simulink model "continuous"  (R2023b)
settings: Solver=FixedStepAuto  StartTime=0.0  StopTime=5  FixedStep=0.01  RelTol=1e-3
InitFcn:
  | clc;clear
  | close all
  | g = [0;2.092];
  | k1 = [-141.9203 -4.5243];
  | k2 = [-101.5134 -3.1941];
  | x0 = [0.4;-10];
settings Model: Creator=IHC  LastModifiedBy=IHC

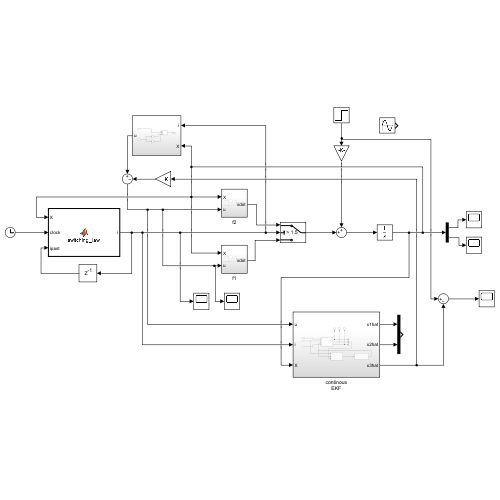
[thumbnail: Simulink's stored preview of the top-level diagram]
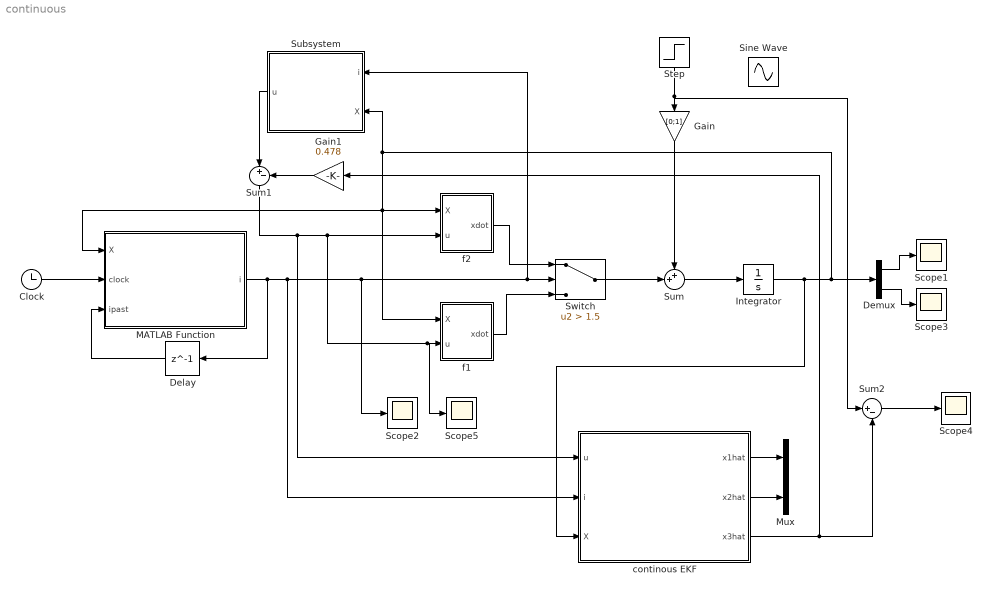
== system continuous ==
  Clock : Clock
  Delay : Delay  DelayLength=1  InitialCondition=2
  Demux : Demux  Outputs=2
  Gain : Gain  Gain=[0;1]
  Gain1 : Gain  Gain=0.478
  Integrator : Integrator  InitialCondition=x0
  MATLAB Function : MATLAB Function  TreatAsAtomicUnit=on
  Mux : Mux  Inputs=2
  Scope{1..5} (5 alike) : Scope
  Sine Wave : Sin  SampleTime=0
  Step : Step  Time=0  After=4  SampleTime=0
  Subsystem : Subsystem
  Sum : Sum  Inputs=++|
  Sum1 : Sum  Inputs=|+-
  Sum2 : Sum  Inputs=|+-
  Switch : Switch  Criteria=u2 > Threshold  Threshold=1.5  SaturateOnIntegerOverflow=off  InputSameDT=off
  continous EKF : Subsystem
  f1 : Subsystem
  f2 : Subsystem
  wires:
  Clock/1 -> MATLAB Function/2(clock)
  Subsystem/1(u) -> Sum1/1
  Demux/1 -> Scope1/1
  Demux/2 -> Scope3/1
  Delay/1 -> MATLAB Function/3(ipast)
  MATLAB Function/1(i) -> Delay/1, continous EKF/2(i), Scope2/1, Subsystem/1(i), Switch/2
  f2/1(xdot) -> Switch/1
  f1/1(xdot) -> Switch/3
  Switch/1 -> Sum/2
  Sum/1 -> Integrator/1
  Gain/1 -> Sum/1
  Step/1 -> Sum2/1, Gain/1
  Integrator/1 -> continous EKF/3(X), Demux/1, MATLAB Function/1(X), f1/1(X), f2/1(X), Subsystem/2(X)
  Sum1/1 -> continous EKF/1(u), Scope5/1, f1/2(u), f2/2(u)
  Sum2/1 -> Scope4/1
  Gain1/1 -> Sum1/2
  continous EKF/3(x3hat) -> Gain1/1, Sum2/2
  continous EKF/1(x1hat) -> Mux/1
  continous EKF/2(x2hat) -> Mux/2

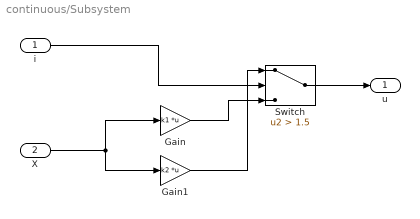
== system continuous/Subsystem ==
  i : Inport
  X : Inport  Port=2
  Gain : Gain  Gain=k1  Multiplication=Matrix(K*u)
  Gain1 : Gain  Gain=k2  Multiplication=Matrix(K*u)
  Switch : Switch  Criteria=u2 > Threshold  Threshold=1.5  SaturateOnIntegerOverflow=off  InputSameDT=off
  u : Outport
  wires:
  Switch/1 -> u/1
  i/1 -> Switch/2
  X/1 -> Gain1/1, Gain/1
  Gain/1 -> Switch/3
  Gain1/1 -> Switch/1

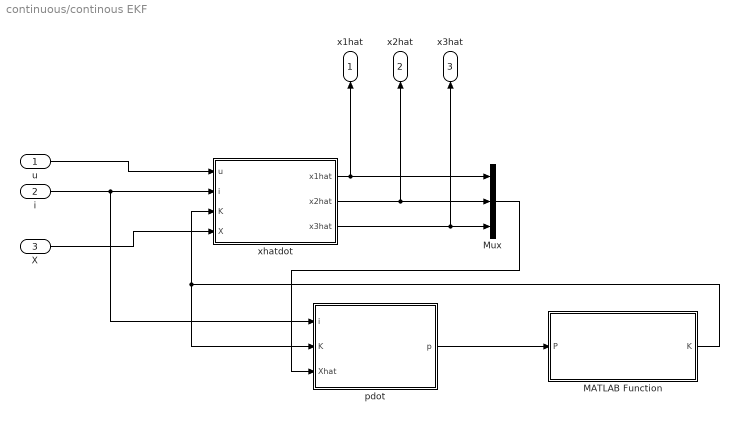
== system continuous/continous EKF ==
  u : Inport
  i : Inport  Port=2
  X : Inport  Port=3
  MATLAB Function : MATLAB Function  TreatAsAtomicUnit=on
  Mux : Mux  Inputs=3
  pdot : Subsystem
  xhatdot : Subsystem
  x1hat : Outport
  x2hat : Outport  Port=2
  x3hat : Outport  Port=3
  wires:
  u/1 -> xhatdot/1(u)
  i/1 -> pdot/1(i), xhatdot/2(i)
  xhatdot/1(x1hat) -> Mux/1, x1hat/1
  xhatdot/2(x2hat) -> Mux/2, x2hat/1
  xhatdot/3(x3hat) -> Mux/3, x3hat/1
  X/1 -> xhatdot/4(X)
  MATLAB Function/1(K) -> pdot/2(K), xhatdot/3(K)
  Mux/1 -> pdot/3(Xhat)
  pdot/1(p) -> MATLAB Function/1(P)

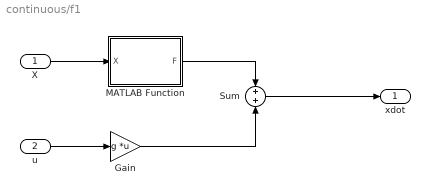
== system continuous/f1 ==
  X : Inport
  u : Inport  Port=2
  Gain : Gain  Gain=g  Multiplication=Matrix(K*u)
  MATLAB Function : MATLAB Function  TreatAsAtomicUnit=on
  Sum : Sum
  xdot : Outport
  wires:
  u/1 -> Gain/1
  X/1 -> MATLAB Function/1(X)
  Gain/1 -> Sum/2
  MATLAB Function/1(F) -> Sum/1
  Sum/1 -> xdot/1

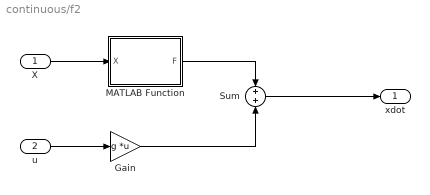
== system continuous/f2 ==
  X : Inport
  u : Inport  Port=2
  Gain : Gain  Gain=g  Multiplication=Matrix(K*u)
  MATLAB Function : MATLAB Function  TreatAsAtomicUnit=on
  Sum : Sum
  xdot : Outport
  wires:
  Sum/1 -> xdot/1
  u/1 -> Gain/1
  MATLAB Function/1(F) -> Sum/1
  Gain/1 -> Sum/2
  X/1 -> MATLAB Function/1(X)

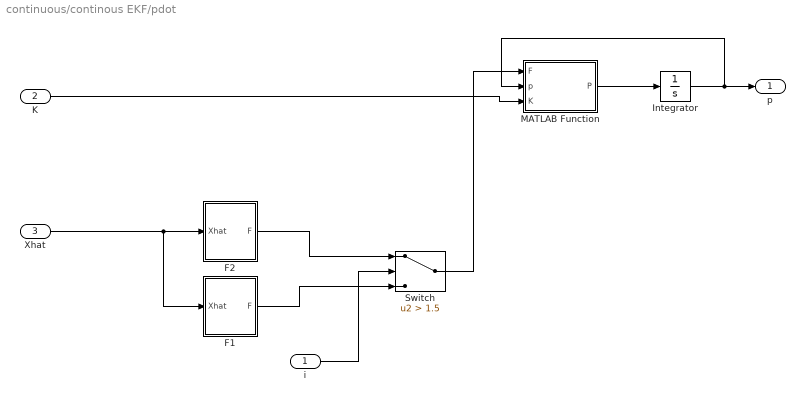
== system continuous/continous EKF/pdot ==
  i : Inport
  K : Inport  Port=2
  Xhat : Inport  Port=3
  F1 : Subsystem
  F2 : Subsystem
  Integrator : Integrator  InitialCondition=diag([0.001,0.001,10])
  MATLAB Function : MATLAB Function  TreatAsAtomicUnit=on
  Switch : Switch  Criteria=u2 > Threshold  Threshold=1.5  SaturateOnIntegerOverflow=off  InputSameDT=off
  p : Outport
  wires:
  F2/1(F) -> Switch/1
  i/1 -> Switch/2
  Integrator/1 -> MATLAB Function/2(p), p/1
  Xhat/1 -> F1/1(Xhat), F2/1(Xhat)
  F1/1(F) -> Switch/3
  MATLAB Function/1(P) -> Integrator/1
  Switch/1 -> MATLAB Function/1(F)
  K/1 -> MATLAB Function/3(K)

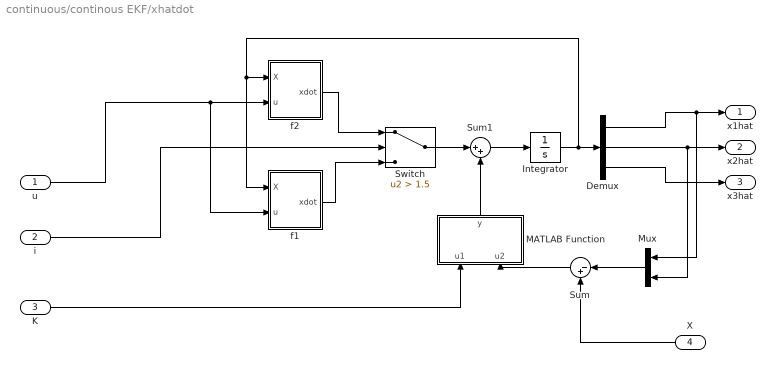
== system continuous/continous EKF/xhatdot ==
  u : Inport
  i : Inport  Port=2
  K : Inport  Port=3
  X : Inport  Port=4
  Demux : Demux  Outputs=3
  Integrator : Integrator  InitialCondition=[x0;0]
  MATLAB Function : MATLAB Function  TreatAsAtomicUnit=on
  Mux : Mux  Inputs=2
  Sum : Sum  Inputs=|-+
  Sum1 : Sum  Inputs=|++
  Switch : Switch  Criteria=u2 > Threshold  Threshold=1.5  SaturateOnIntegerOverflow=off  InputSameDT=off
  f1 : Subsystem
  f2 : Subsystem
  x1hat : Outport
  x2hat : Outport  Port=2
  x3hat : Outport  Port=3
  wires:
  Demux/2 -> Mux/2, x2hat/1
  Demux/3 -> x3hat/1
  f1/1(xdot) -> Switch/3
  f2/1(xdot) -> Switch/1
  u/1 -> f1/2(u), f2/2(u)
  i/1 -> Switch/2
  Demux/1 -> Mux/1, x1hat/1
  Integrator/1 -> f1/1(X), f2/1(X), Demux/1
  Switch/1 -> Sum1/1
  Sum1/1 -> Integrator/1
  X/1 -> Sum/2
  Mux/1 -> Sum/1
  MATLAB Function/1(y) -> Sum1/2
  Sum/1 -> MATLAB Function/2(u2)
  K/1 -> MATLAB Function/1(u1)

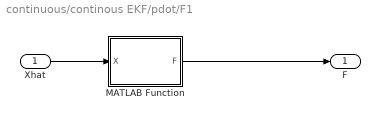
== system continuous/continous EKF/pdot/F1 ==
  Xhat : Inport
  MATLAB Function : MATLAB Function  TreatAsAtomicUnit=on
  F : Outport
  wires:
  Xhat/1 -> MATLAB Function/1(X)
  MATLAB Function/1(F) -> F/1

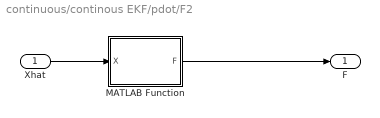
== system continuous/continous EKF/pdot/F2 ==
  Xhat : Inport
  MATLAB Function : MATLAB Function  TreatAsAtomicUnit=on
  F : Outport
  wires:
  Xhat/1 -> MATLAB Function/1(X)
  MATLAB Function/1(F) -> F/1

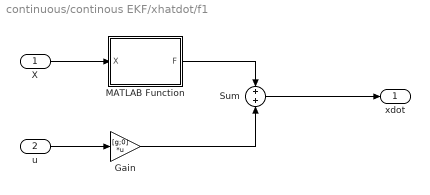
== system continuous/continous EKF/xhatdot/f1 ==
  X : Inport
  u : Inport  Port=2
  Gain : Gain  Gain=[g;0]  Multiplication=Matrix(K*u)
  MATLAB Function : MATLAB Function  TreatAsAtomicUnit=on
  Sum : Sum
  xdot : Outport
  wires:
  u/1 -> Gain/1
  X/1 -> MATLAB Function/1(X)
  Gain/1 -> Sum/2
  MATLAB Function/1(F) -> Sum/1
  Sum/1 -> xdot/1

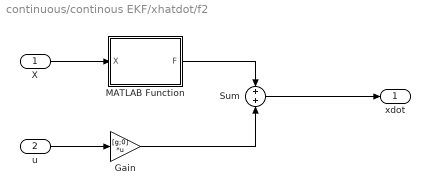
== system continuous/continous EKF/xhatdot/f2 ==
  X : Inport
  u : Inport  Port=2
  Gain : Gain  Gain=[g;0]  Multiplication=Matrix(K*u)
  MATLAB Function : MATLAB Function  TreatAsAtomicUnit=on
  Sum : Sum
  xdot : Outport
  wires:
  Sum/1 -> xdot/1
  u/1 -> Gain/1
  MATLAB Function/1(F) -> Sum/1
  Gain/1 -> Sum/2
  X/1 -> MATLAB Function/1(X)

== matlab function continuous/f2/MATLAB Function ==
  data: X input; F output
function F = fcn(X)
x1 = X(1);
x2 = X(2);
alpha = -7.2*10^10*(x1+0.5)*exp(-8750/(x2+350))+0.5;
beta = 1.506*10^13*(x1+0.5)*exp(-8750/(x2+350))-104.6;
f1=-2*x1+alpha;
f2 =-4.092*x2+beta;
F=[f1;f2];
end

== matlab function continuous/f1/MATLAB Function ==
  data: X input; F output
function F = fcn(X)
x1 = X(1);
x2 = X(2);
alpha = -7.2*10^10*(x1+0.5)*exp(-8750/(x2+350))+0.5;
beta = 1.506*10^13*(x1+0.5)*exp(-8750/(x2+350))-104.6;
f1=-0.5*x1+alpha;
f2 =-2.592*x2+beta;
F=[f1;f2];
end

== matlab function continuous/MATLAB Function ==
  data: X input; i output; clock input; ipast input
function i = switching_law(X,clock,ipast)
x1 = X(1);
x2 = X(2);
g = [0;2.092];
vx1 = zeros(1,2);
vx2 = zeros(1,2);

vx1(1,1) = [6175.531 135.679]*X;
vx1(1,2) = [135.679 4.3253]*X;
vx2(1,1) = [3590.3982 97.0491]*X;
vx2(1,2) = [97.0491 3.0536]*X;
alpha = -7.2*10^10*(x1+0.5)*exp(-8750/(x2+350))+0.5;
beta = 1.506*10^13*(x1+0.5)*exp(-8750/(x2+350))-104.6;
f1 = [-0.5*x1+alpha;-2.592*x2+beta];
f2 = [-2*x1+alpha;-4.092*x2+beta]; 
a = vx1*f1 - (1/4)*vx1*g*g'*vx1';
b = vx2*f2 - (1/4)*vx2*g*g'*vx2';

if mod(clock,0.1) == 0
    if b < a
        i = 2;
    else
        i = 1;
    end
else
    i = ipast;
end
end

== matlab function continuous/continous EKF/MATLAB Function ==
  data: P input; K output
function K = kalman_filter_gain(P)
    
    H = [1 0 0;
         0  1  0];
    R = 1e-5*eye(2);
    K = P*H'*R^-1;
end

== matlab function continuous/continous EKF/pdot/MATLAB Function ==
  data: F input; P output; p input; K input
function P = fcn(F,p,K)
Q = diag([0.001,0.001,0.001]);
H = [1 0 0;0 1 0];
P = F*p+p*F'-K*H*p+Q;
end

== matlab function continuous/continous EKF/xhatdot/f1/MATLAB Function ==
  data: X input; F output
function F = fcn(X)
x1 = X(1);
x2 = X(2);
x3 = X(3);
alpha = -7.2*10^10*(x1+0.5)*exp(-8750/(x2+350))+0.5;
beta = 1.506*10^13*(x1+0.5)*exp(-8750/(x2+350))-104.6;
f1=-0.5*x1+alpha;
f2 =-2.592*x2+beta+x3;
F=[f1;f2;0];
end

== matlab function continuous/continous EKF/xhatdot/f2/MATLAB Function ==
  data: X input; F output
function F = fcn(X)
x1 = X(1);
x2 = X(2);
x3 = X(3);
alpha = -7.2*10^10*(x1+0.5)*exp(-8750/(x2+350))+0.5;
beta = 1.506*10^13*(x1+0.5)*exp(-8750/(x2+350))-104.6;
f1=-2*x1+alpha;
f2 =-4.092*x2+beta+x3;
F=[f1;f2;0];
end

== matlab function continuous/continous EKF/pdot/F2/MATLAB Function ==
  data: X input; F output
function F = fcn(X)
x1 = X(1);
x2 = X(2);
x3 = X(3);

F = [- 72000000000*exp(-8750/(x2 + 350)) - 2,                -(8750*exp(-8750/(x2 + 350))*(72000000000*x1 + 36000000000))/(x2 + 350)^2, 0;
   15060000000000*exp(-8750/(x2 + 350)), (8750*exp(-8750/(x2 + 350))*(15060000000000*x1 + 7530000000000))/(x2 + 350)^2 - 1023/250, 1;
                                      0,                                                                                        0, 0];
 
end

== matlab function continuous/continous EKF/pdot/F1/MATLAB Function ==
  data: X input; F output
function F = fcn(X)
x1 = X(1);
x2 = X(2);
x3 = X(3);

F = [- 72000000000*exp(-8750/(x2 + 350)) - 1/2,               -(8750*exp(-8750/(x2 + 350))*(72000000000*x1 + 36000000000))/(x2 + 350)^2, 0;
     15060000000000*exp(-8750/(x2 + 350)), (8750*exp(-8750/(x2 + 350))*(15060000000000*x1 + 7530000000000))/(x2 + 350)^2 - 324/125, 1;
                                        0,                                                                                       0, 0];
 
end

== matlab function continuous/continous EKF/xhatdot/MATLAB Function ==
  data: u1 input; y output; u2 input
function y = fcn(u1,u2)

y = u1*u2;
end
